simulink model "JAWS_vessel"  (R2021a)
settings: Solver=VariableStepAuto  StartTime=0.0  StopTime=10.0  RelTol=1e-3
libraries: mssSimulink x4
settings Model: Creator=premr  LastModifiedBy=premr

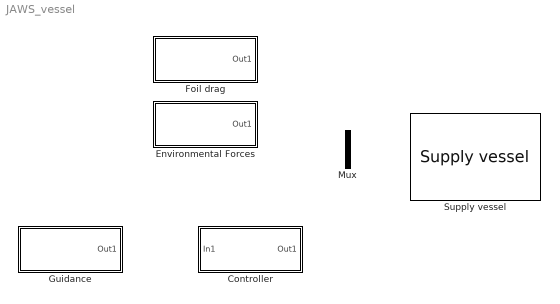
== system JAWS_vessel ==
  Controller : Subsystem
  Environmental Forces : Subsystem
  Foil drag : Subsystem
  Guidance : Subsystem
  Mux : Mux  Inputs=3
  Supply vessel : mssSimulink/Marine craft models/Supply vessel  D=[5.0242e4 0 0; 0 2.7229e5 -4.3933e6; 0 -4.3933e6 4.1894e8]  Minv=inv( [5.3122e6 0 0; 0 8.2831e6 0; 0 0 3.7454e9] )

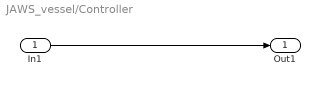
== system JAWS_vessel/Controller ==
  In1 : Inport
  Out1 : Outport
  wires:
  In1/1 -> Out1/1

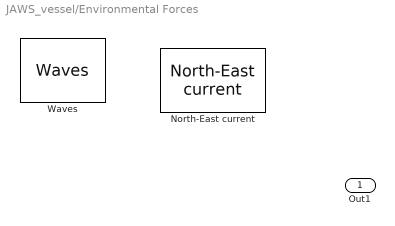
== system JAWS_vessel/Environmental Forces ==
  North-East current : mssSimulink/Environment/Current/North-East current  SystemSampleTime=-1  VariantActivationTime=update diagram  Latency=0  AutoFrameSizeCalculation=off
  Waves : mssSimulink/Environment/Waves/Waves  spectrum_type=ITTC  disp_flag=on  plot_spectrum=off  plot_realization=off  hs=0.8  omega_peak=0  psi_mean=0  gamma=-1  spread=2  depth=inf  nfreq=20  ndir=10  energylim=0.005  freq_cutoff=3  dir_cutoff=0  rand_seed=123  rand_freq=on  rand_dir=on  Zeta_a=0  Omega=0  Phase=0  Wavenum=0  Psi=0
  Out1 : Outport
  wires:
  ? -> Out1/1

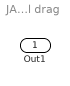
== system JAWS_vessel/Foil drag ==
  Out1 : Outport
  wires:
  ? -> Out1/1

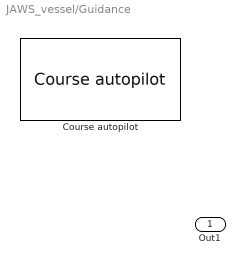
== system JAWS_vessel/Guidance ==
  Course autopilot : mssSimulink/Control/Autopilots/Course autopilot  wn=1.2  zeta=1  T_nomoto=0.5  m=37.1
  Out1 : Outport
  wires:
  ? -> Out1/1
